simulink model "Quaternions_Method_merge"  (R2021b)
settings: Solver=VariableStepAuto  StartTime=0.0  StopTime=Time  MinStep=1e-3  RelTol=1e-13  AbsTol=1e-8
undefined symbols (not defined in the file): a, c, e, f_mag, H_0, i, magnitude, MB, muP, omega_0, p_acc, RD, RS_MB, RS_SP, SP, theta0, w_E
libraries: matrix_library x10, vrlib x4, simulink_extras x1
(part 1 of 3)
settings Model: Creator=dario  LastModifiedBy=hp
settings SolverCC: ZeroCrossControl=DisableAll  ZeroCrossAlgorithm=Adaptive  AlgebraicLoopSolver=TrustRegion
settings DebuggingCC: IgnoredZcDiagnostic=none

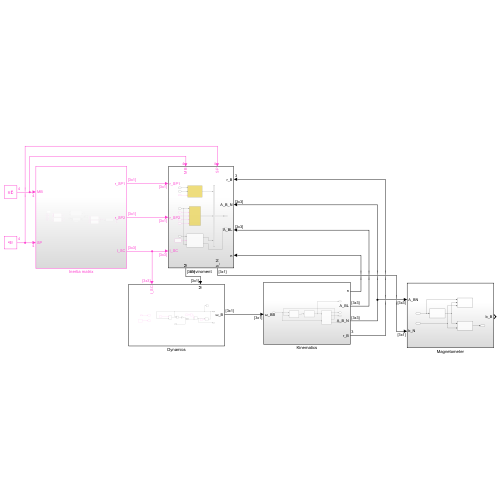
[thumbnail: Simulink's stored preview of the top-level diagram]
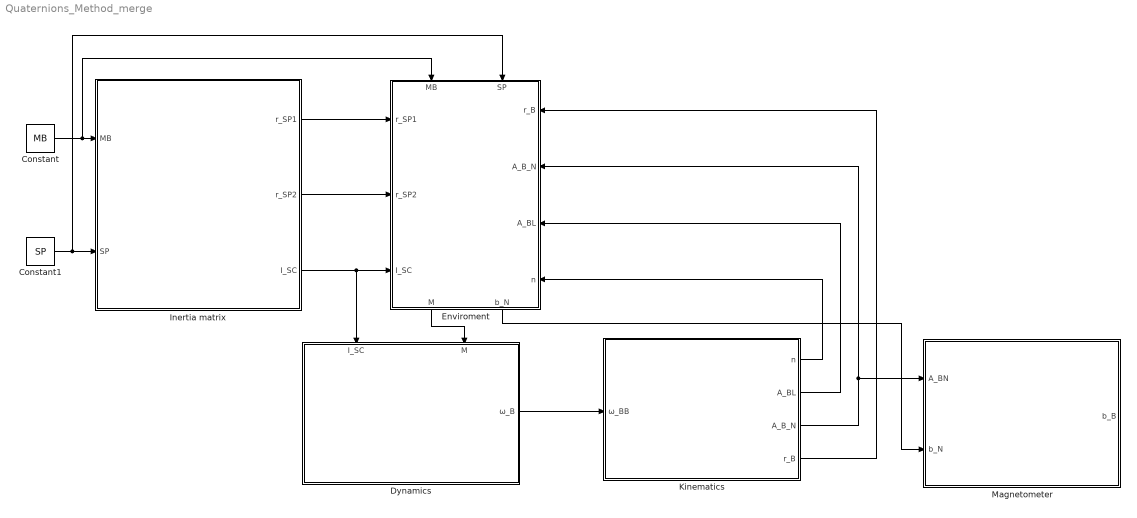
== system Quaternions_Method_merge ==
  Constant : Constant  Value=MB
  Constant1 : Constant  Value=SP
  Dynamics : Subsystem
      settings: PortSchema="{\"entries\":[{\"content\":{\"sides\":[{\"content\":{\"connectorIds\":[]},\"type\":\"ConnectorPlacement.EquallySpacedRectSide\",\"uuid\":\"0fb0fd28-732a-45b7-951f-4b0b2306202c\"},{\"content\":{\"connectorIds\":[\"Out1\"],\"side\":\"RIGHT\"},\"type\":\"ConnectorPlacement.EquallySpacedRectSide\",\"uuid\":\"160a6d95-5e8b-4088-9ac4-372e2ef53b1e\"},{\"content\":{\"connectorIds\":[\"In1\",\"In2\"],\"side\":\"TOP\"},\"type\":\"ConnectorPlacement.EquallySpacedRectSide\",\"uuid\":\"bc0d773d-9b3c-40c2-804a-fc9efd6e220c\"}]},\"type\":\"ConnectorPlacement.EquallySpacedConnector\",\"uuid\":\"1f85a25c-c8d4-4d9d-9994-483d99135538\"}],\"packageUris\":[\"http://schema.mathworks.com/mf0/Connector/R2020b\"],\"version\":\"1.0\"}"
  Enviroment : Subsystem
      settings: PortSchema="{\"entries\":[{\"content\":{\"sides\":[{\"content\":{\"connectorIds\":[\"In1\",\"In2\"]},\"type\":\"ConnectorPlacement.EquallySpacedRectSide\",\"uuid\":\"77a65197-c5ef-4c05-af97-bd670bb59a1b\"},{\"content\":{\"connectorIds\":[\"Out1\",\"Out2\"],\"side\":\"RIGHT\"},\"type\":\"ConnectorPlacement.EquallySpacedRectSide\",\"uuid\":\"f4905732-994b-44e8-915f-1f1165b6d340\"},{\"content\":{\"connectorIds\":[\"In3\",\"In4\",\"In5\"],\"side\":\"TOP\"},\"type\":\"ConnectorPlacement.EquallySpacedRectSide\",\"uuid\":\"dbb628bc-072b-4daa-a580-a056bf799753\"},{\"content\":{\"connectorIds\":[\"In6\",\"In7\",\"In8\",\"In9\"],\"side\":\"BOTTOM\"},\"type\":\"ConnectorPlacement.EquallySpacedRectSide\",\"uuid\":\"e6af6235-b92e-4098-9bbc-91b77f168ead\"}]},\"type\":\"ConnectorPlacement.EquallySpacedConnector\",\"uuid\":\"a4645f0d-8f51-4ba7-9ec5-d423e83ccc17\"}],\"packageUris\":[\"http://schema.mathworks.com/mf0/Connector/R2020b\"],\"version\":\"1.0\"}"
  Inertia matrix : Subsystem
  Kinematics : Subsystem
  Magnetometer : Subsystem
  wires:
  Enviroment/1(M) -> Dynamics/2(M)
  Kinematics/2(A_BL) -> Enviroment/8(A_BL)
  Dynamics/1(ω_B) -> Kinematics/1(ω_BB)
  Kinematics/1(n) -> Enviroment/9(n)
  Kinematics/3(A_B_N) -> Magnetometer/1(A_BN), Enviroment/7(A_B_N)
  Constant/1 -> Inertia matrix/1(MB), Enviroment/1(MB)
  Constant1/1 -> Inertia matrix/2(SP), Enviroment/2(SP)
  Inertia matrix/1(r_SP1) -> Enviroment/3(r_SP1)
  Inertia matrix/2(r_SP2) -> Enviroment/4(r_SP2)
  Inertia matrix/3(I_SC) -> Dynamics/1(I_SC), Enviroment/5(I_SC)
  Kinematics/4(r_B) -> Enviroment/6(r_B)
  Enviroment/2(b_N) -> Magnetometer/2(b_N)

== system Quaternions_Method_merge/Dynamics ==
  I_SC : Inport
  M : Inport  Port=2
  Constant7 : Constant  Value=omega_0
  Cross Product : vrlib/Utilities/Cross Product
  Gain5 : Gain  Gain=-1
  Integrator4 : Integrator  InitialConditionSource=external  InitialCondition=omega_0
  Product6 : Product  Multiplication=Matrix(*)
  Product7 : Product  Multiplication=Matrix(*)
  Reciprocal : Product  Inputs=/  Multiplication=Matrix(*)
  Scope : Scope
  Sum2 : Sum
  Terminator : Terminator
  ω_B : Outport
  wires:
  Sum2/1 -> Product7/2
  Product6/1 -> Cross Product/2
  Product7/1 -> Terminator/1, Integrator4/1
  Cross Product/1 -> Gain5/1
  Gain5/1 -> Sum2/1
  Integrator4/1 -> Scope/1, Cross Product/1, Product6/2, ω_B/1
  I_SC/1 -> [I_SC]
  [I_SC] -> Product6/1
  [I_SC] -> Reciprocal/1
  Reciprocal/1 -> Product7/1
  Constant7/1 -> [w_0]
  [w_0] -> Integrator4/2
  M/1 -> Sum2/2

== system Quaternions_Method_merge/Enviroment ==
  MB : Inport
  SP : Inport  Port=2
  r_SP1 : Inport  Port=3
  r_SP2 : Inport  Port=4
  I_SC : Inport  Port=5
  r_B : Inport  Port=6
  A_B_N : Inport  Port=7
  A_BL : Inport  Port=8
  n : Inport  Port=9
  Constant : Constant  Value=6371.2*1e3
  Gravity Gradient : Subsystem
  "Magnetic torque " : Subsystem
  Solar Radiation Perturbation : Subsystem
  Sum : Sum  Inputs=+|+|+
  M : Outport
  b_N : Outport  Port=2
  wires:
  A_BL/1 -> Gravity Gradient/1(A_BL)
  n/1 -> Gravity Gradient/2(n)
  A_B_N/1 -> "Magnetic torque "/3(A_B_N), Solar Radiation Perturbation/1(A_B_N)
  MB/1 -> Solar Radiation Perturbation/2(MB)
  SP/1 -> Solar Radiation Perturbation/3(SP)
  r_SP1/1 -> Solar Radiation Perturbation/4(r_SP1)
  r_SP2/1 -> Solar Radiation Perturbation/5(r_SP2)
  Sum/1 -> M/1
  Gravity Gradient/1(M_GG) -> Sum/1
  Solar Radiation Perturbation/1(M_SRP) -> Sum/2
  I_SC/1 -> Gravity Gradient/3(I_SC)
  "Magnetic torque "/1(M) -> Sum/3
  r_B/1 -> "Magnetic torque "/1(r_B)
  Constant/1 -> "Magnetic torque "/2(R)
  "Magnetic torque "/2(b_N) -> b_N/1

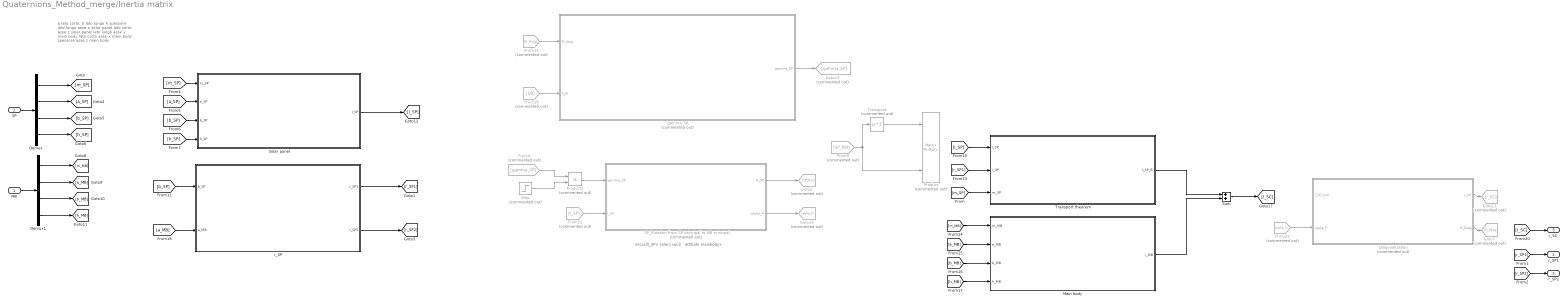
== system Quaternions_Method_merge/Inertia matrix ==
  note: arcos(S_B*n solary)-pi/2 - attitude mainbodyx
  note: a lato corto, b lato lungo h spessore
      | lato lungo asse x solar panel
      | lato corto asse z solar panel
      | lato lungo asse y main body
      | lato corto asse x main body
      | spessore asse z main body
  MB : Inport
  SP : Inport  Port=2
  Demux : Demux
  Demux1 : Demux
  Diagonalization : Subsystem  Commented=on
  From12 : From  Commented=on  GotoTag=R_Diag
  From19 : From  Commented=on  GotoTag=SB
  From21 : From  Commented=on  GotoTag=I_SP
  From22 : From  Commented=on  GotoTag=alpha_P
  From8 : From  Commented=on  GotoTag=gamma_SP
  From9 : From  Commented=on  GotoTag=SP_Rot
  Goto13 : Goto  Commented=on  GotoTag=I_SC
  Goto14 : Goto  Commented=on  GotoTag=gamma_SP
  Goto16 : Goto  Commented=on  GotoTag=alpha_P
  Goto2 : Goto  Commented=on  GotoTag=SP_Rot
  Goto7 : Goto  Commented=on  GotoTag=R_Diag
  Main body : Subsystem
  Product : Product  Commented=on  Inputs=3  Multiplication=Matrix(*)
  Product1 : Product  Commented=on
  SP_Rotation from SP principal to MB principal : Subsystem  Commented=on
  Solar panel : Subsystem
  Step : Step  Commented=on  Time=1e-3  SampleTime=0
  Sum : Sum
  Transport theorem : Subsystem
  Transpose : Math  Commented=on  Operator=transpose  SaturateOnIntegerOverflow=on
  gamma_SP : Subsystem  Commented=on
  r_SP : Subsystem
  r_SP1 : Outport
  r_SP2 : Outport  Port=2
  I_SC : Outport  Port=3
  wires:
  MB/1 -> Demux1/1
  Demux/1 -> [m_SP]
  SP_Rotation from SP principal to MB principal/1(R_SP) -> Goto2/1
  Transpose/1 -> Product/1
  Transport theorem/1(I_SP_B) -> Sum/1
  [r_SP1] -> Transport theorem/2(r_SP)
  Main body/1(I_MB) -> Sum/2
  [m_SP] -> Transport theorem/3(m_SP)
  r_SP/1(r_SP1) -> [r_SP1]
  [r_SP1] -> r_SP1/1
  [r_SP2] -> r_SP2/1
  r_SP/2(r_SP2) -> [r_SP2]
  Demux/2 -> [a_SP]
  Demux/3 -> [b_SP]
  Demux/4 -> [h_SP]
  [a_SP] -> Solar panel/2(a_SP)
  [b_SP] -> Solar panel/3(b_SP)
  [m_SP] -> Solar panel/1(m_SP)
  [h_SP] -> Solar panel/4(h_SP)
  From9/1 -> Transpose/1, Product/3
  [b_SP] -> r_SP/1(b_SP)
  Demux1/4 -> [h_MB]
  Demux1/3 -> [b_MB]
  Demux1/2 -> [a_MB]
  Demux1/1 -> [m_MB]
  [m_MB] -> Main body/1(m_MB)
  [a_MB] -> Main body/2(a_MB)
  [b_MB] -> Main body/3(b_MB)
  [h_MB] -> Main body/4(h_MB)
  [a_MB] -> r_SP/2(a_MB)
  Solar panel/1(I_SP) -> [I_SP]
  Product1/1 -> SP_Rotation from SP principal to MB principal/1(gamma_SP)
  From8/1 -> Product1/1
  Step/1 -> Product1/2
  SP/1 -> Demux/1
  Diagonalization/2(R_Diag) -> Goto7/1
  From12/1 -> gamma_SP/1(R_diag)
  From19/1 -> gamma_SP/2(S_B)
  Diagonalization/1(I_SC) -> Goto13/1
  [I_SC] -> I_SC/1
  gamma_SP/1(gamma_SP) -> Goto14/1
  From21/1 -> SP_Rotation from SP principal to MB principal/2(I_SP)
  SP_Rotation from SP principal to MB principal/2(alpha_P) -> Goto16/1
  From22/1 -> Diagonalization/2(alpha_P)
  [I_SP] -> Transport theorem/1(I_SP)
  Sum/1 -> [I_SC]

== system Quaternions_Method_merge/Kinematics ==
  ω_BB : Inport
  Creazione Matrice A_BN : Subsystem
  Creazione quaternione : Subsystem
  Relative_Attitude : Subsystem
  n : Outport
  A_BL : Outport  Port=2
  A_B_N : Outport  Port=3
  r_B : Outport  Port=4
  wires:
  Creazione Matrice A_BN/1(A_BN) -> A_B_N/1, Relative_Attitude/1(A_BN)
  ω_BB/1 -> Creazione quaternione/1(ω_BB), Relative_Attitude/2(ω_BB)
  Creazione quaternione/1(q_normalizzato) -> Creazione Matrice A_BN/1(q_normalizzato)
  Relative_Attitude/1(A_BL) -> A_BL/1
  Relative_Attitude/2(n) -> n/1
  Relative_Attitude/3(A_L/N) -> Creazione quaternione/2(A_LN)
  Relative_Attitude/4(r_B) -> r_B/1

== system Quaternions_Method_merge/Magnetometer ==
  A_BN : Inport
  b_N : Inport  Port=2
  Compute b_B : Subsystem
  Difference between model and reality : Subsystem
  "Magnetometer " : Subsystem
  b_B : Outport
  wires:
  "Magnetometer "/1(A_BN*) -> Compute b_B/1(A_BN*), Difference between model and reality/2(A_BN*)
  A_BN/1 -> Difference between model and reality/1(A_BN), "Magnetometer "/1(A_BN)
  b_N/1 -> Compute b_B/2(b_N), Difference between model and reality/3(b_N)
  Compute b_B/1(b_B) -> b_B/1

== system Quaternions_Method_merge/Enviroment/Gravity Gradient ==
  A_BL : Inport
  n : Inport  Port=2
  I_SC : Inport  Port=3
  Constant1 : Constant  Value=[1; 0; 0]
  Demux : Demux  Outputs=9
  Demux2 : Demux  Outputs=3
  Gain1 : Gain  Gain=3
  Matrix Multiply : Product  Multiplication=Matrix(*)
  Mux1 : Mux  Inputs=3
  Product{,4..11} (9 alike) : Product
  Reshape : Reshape  OutputDimensionality=Column vector (2-D)
  Reshape1 : Reshape  OutputDimensionality=Column vector (2-D)
  Square1 : Math  Operator=square  SaturateOnIntegerOverflow=on
  Sum3 : Sum  Inputs=|+|-|
  Sum4 : Sum  Inputs=|+|-|
  Sum5 : Sum  Inputs=|+|-|
  Terminator{,1..5} (6 alike) : Terminator
  M_GG : Outport
  wires:
  A_BL/1 -> Matrix Multiply/1
  Constant1/1 -> Matrix Multiply/2
  Matrix Multiply/1 -> Demux2/1
  Demux2/1 -> Product4/1, Product/1  "c1"
  Demux2/3 -> Product5/2, Product4/2  "c3"
  Demux2/2 -> Product5/1, Product/2  "c2"
  Demux/9 -> Sum4/2, Sum3/1  "Iz"
  Demux/5 -> Sum5/1, Sum3/2  "Iy"
  Demux/1 -> Sum5/2, Sum4/1  "Ix"
  n/1 -> Square1/1
  Square1/1 -> Gain1/1
  Product5/1 -> Product6/1
  Gain1/1 -> Product9/2, Product7/2, Product6/2
  Product4/1 -> Product7/1
  Product/1 -> Product9/1
  Sum3/1 -> Product8/1
  Product6/1 -> Product8/2
  Product7/1 -> Product10/1
  Sum4/1 -> Product10/2
  Sum5/1 -> Product11/2
  Product9/1 -> Product11/1
  Product10/1 -> Mux1/2
  Product8/1 -> Mux1/1
  Product11/1 -> Mux1/3
  Mux1/1 -> Reshape/1
  Reshape/1 -> M_GG/1
  I_SC/1 -> Reshape1/1
  Demux/2 -> Terminator/1
  Demux/3 -> Terminator1/1
  Demux/4 -> Terminator2/1
  Demux/6 -> Terminator3/1
  Demux/7 -> Terminator4/1
  Demux/8 -> Terminator5/1
  Reshape1/1 -> Demux/1

== system Quaternions_Method_merge/Enviroment/Magnetic torque  ==
  r_B : Inport
  R : Inport  Port=2
  A_B_N : Inport  Port=3
  Creation of parasitic torque : Subsystem
  Magnetic torque in body frame : Subsystem
  Matrix Multiply : Product  Multiplication=Matrix(*)
  Product : Product
  M : Outport
  b_N : Outport  Port=2
  wires:
  R/1 -> Magnetic torque in body frame/3(R)
  A_B_N/1 -> Magnetic torque in body frame/1(A_B_N), Matrix Multiply/1
  Magnetic torque in body frame/1(b_B) -> Product/1
  Creation of parasitic torque/1(m) -> Product/2
  Product/1 -> M/1
  Matrix Multiply/1 -> Magnetic torque in body frame/2(r_N)
  r_B/1 -> Matrix Multiply/2
  Magnetic torque in body frame/2(b_N) -> b_N/1

== system Quaternions_Method_merge/Enviroment/Solar Radiation Perturbation ==
  A_B_N : Inport
  MB : Inport  Port=2
  SP : Inport  Port=3
  r_SP1 : Inport  Port=4
  r_SP2 : Inport  Port=5
  Force : Subsystem
  Normalize Vector : vrlib/Utilities/Normalize Vector  maxzero=0
  Sum forces : Subsystem
      settings: PortSchema="{\"entries\":[{\"content\":{\"sides\":[{\"content\":{\"connectorIds\":[\"In1\",\"In2\",\"In3\",\"In4\",\"In5\",\"In6\",\"In7\"]},\"type\":\"ConnectorPlacement.EquallySpacedRectSide\",\"uuid\":\"5acb7d4f-0337-4224-9758-4598a3a00165\"},{\"content\":{\"connectorIds\":[\"Out1\"],\"side\":\"RIGHT\"},\"type\":\"ConnectorPlacement.EquallySpacedRectSide\",\"uuid\":\"e6f98c05-9b5f-4378-b9e9-dabff353d596\"},{\"content\":{\"connectorIds\":[],\"side\":\"TOP\"},\"type\":\"ConnectorPlacement.EquallySpacedRectSide\",\"uuid\":\"88e90ea7-7ab4-48d4-8e3b-8712b3a0b993\"},{\"content\":{\"connectorIds\":[\"In8\"],\"side\":\"BOTTOM\"},\"type\":\"ConnectorPlacement.EquallySpacedRectSide\",\"uuid\":\"ececea6a-2c27-462e-a638-503b4beb3cbf\"}]},\"type\":\"ConnectorPlacement.EquallySpacedConnector\",\"uuid\":\"86da1db6-5ce7-4d9e-9b5c-c43957a7360d\"}],\"packageUris\":[\"http://schema.mathworks.com/mf0/Connector/R2020b\"],\"version\":\"1.0\"}"
  Sun position body : Subsystem
  normali SP1 : Constant  Value=[0 1 0; 0 -1 0; 0 1 0; 0 -1 0]
  M_SRP : Outport
  tag scope: S_B=global
  wires:
  A_B_N/1 -> Sun position body/1(A_B_N)
  Sun position body/1(S_B) -> Normalize Vector/1
  Normalize Vector/1 -> [S_B], Force/1(SB)
  Force/3(A_MB) -> Sum forces/5(A_MB)
  Force/1(F_MB) -> Sum forces/3(F_MB)
  normali SP1/1 -> Force/2(N_SP)
  r_SP1/1 -> Sum forces/1(r_SP1)
  r_SP2/1 -> Sum forces/2(r_SP2)
  Force/5(prodscal_SP) -> Sum forces/7(prodscal_SP (tra norm e sun direction))
  Force/4(prodsca_MB) -> Sum forces/6(prodscal_MB(tra norm e sun direction))
  Sum forces/1(M_SRP) -> M_SRP/1
  MB/1 -> [MB]
  SP/1 -> [SP]
  [MB] -> Force/3(MB)
  [SP] -> Force/4(SP)
  [MB] -> Sum forces/8(MB)
  Force/2(F_SP) -> Sum forces/4(F_SP)

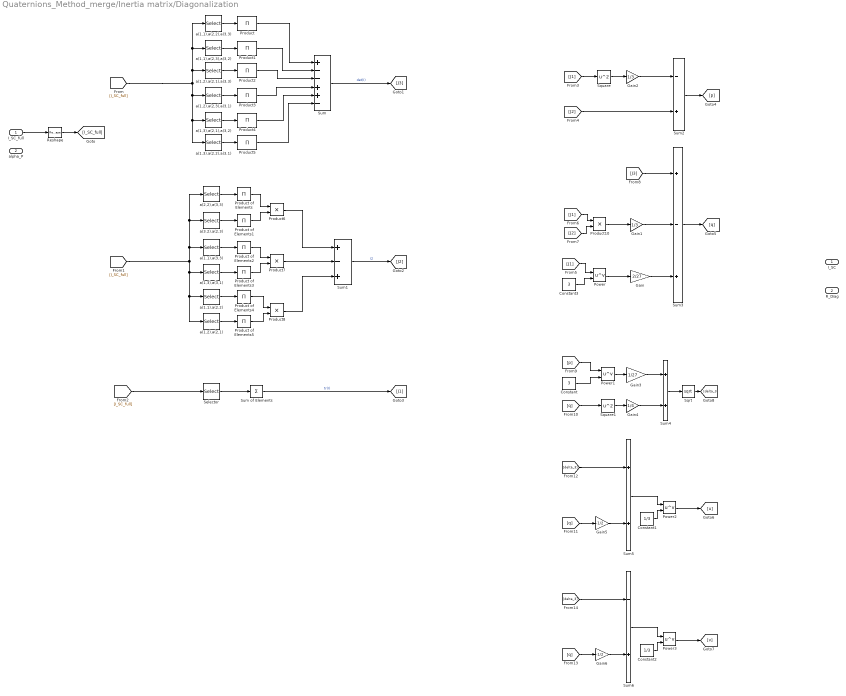
== system Quaternions_Method_merge/Inertia matrix/Diagonalization ==
  I_SC_full : Inport
  alpha_P : Inport  Port=2
  Constant : Constant  Value=3
  Constant1 : Constant  Value=1/3
  Constant2 : Constant  Value=1/3
  Constant3 : Constant  Value=3
  Gain : Gain  Gain=2/27
  Gain1 : Gain  Gain=1/3
  Gain2 : Gain  Gain=1/3
  Gain3 : Gain  Gain=1/27
  Gain4 : Gain  Gain=1/4
  Gain5 : Gain  Gain=-1/2
  Gain6 : Gain  Gain=-1/2
  Power{,1..3} (4 alike) : Math  Operator=pow  SaturateOnIntegerOverflow=on
  Product{,1..5} (6 alike) : Product  Inputs=1  SaturateOnIntegerOverflow=on  OutDataTypeStr=Inherit: Same as first input
  Product of Elements{,1..5} (6 alike) : Product  Inputs=*
  Product{6..8,10} (4 alike) : Product
  Reshape : Reshape  OutputDimensionality=Column vector (2-D)
  Selector : Selector  InputPortWidth=9  IndexOptions=Index vector (dialog)  Indices=[1 5 9]  OutputSizes=1
  Sqrt : Sqrt  SaturateOnIntegerOverflow=on
  Square : Math  Operator=square  SaturateOnIntegerOverflow=on
  Square1 : Math  Operator=square  SaturateOnIntegerOverflow=on
  Sum : Sum  Inputs=+--++-  SaturateOnIntegerOverflow=on
  Sum of Elements : Sum  Inputs=+
  Sum1 : Sum  Inputs=+-+
  Sum2 : Sum  Inputs=-+
  Sum3 : Sum  Inputs=+-+
  Sum4 : Sum
  Sum5 : Sum
  Sum6 : Sum  Inputs=-+
  a(1,1),a(2,2) : Selector  InputPortWidth=9  IndexOptions=Index vector (dialog)  Indices=[1 3]  OutputSizes=1
  a(1,1),a(2,2),a(3,3) : Selector  InputPortWidth=9  IndexOptions=Index vector (dialog)  Indices=[1 5 9]  OutputSizes=1
  a(1,1),a(2,3),a(3,2) : Selector  InputPortWidth=9  IndexOptions=Index vector (dialog)  Indices=[1 6 8]  OutputSizes=1
  a(1,2),a(2,1) : Selector  InputPortWidth=9  IndexOptions=Index vector (dialog)  Indices=[1 3]  OutputSizes=1
  a(1,2),a(2,1),a(3,3) : Selector  InputPortWidth=9  IndexOptions=Index vector (dialog)  Indices=[2 4 9]  OutputSizes=1
  a(1,2),a(2,3),a(3,1) : Selector  InputPortWidth=9  IndexOptions=Index vector (dialog)  Indices=[3 4 8]  OutputSizes=1
  a(1,3),a(2,1),a(3,2) : Selector  InputPortWidth=9  IndexOptions=Index vector (dialog)  Indices=[2 6 7]  OutputSizes=1
  a(1,3),a(2,2),a(3,1) : Selector  InputPortWidth=9  IndexOptions=Index vector (dialog)  Indices=[3 5 7]  OutputSizes=1
  a(1,3),a(3,1) : Selector  InputPortWidth=9  IndexOptions=Index vector (dialog)  Indices=[1 3]  OutputSizes=1
  a(1.1),a(3,3) : Selector  InputPortWidth=9  IndexOptions=Index vector (dialog)  Indices=[1 3]  OutputSizes=1
  a(2,2),a(3,3) : Selector  InputPortWidth=9  IndexOptions=Index vector (dialog)  Indices=[5 9]  OutputSizes=1
  a(3.2),a(2,3) : Selector  InputPortWidth=9  IndexOptions=Index vector (dialog)  Indices=[6 8]  OutputSizes=1
  I_SC : Outport
  R_Diag : Outport  Port=2
  wires:
  [I_SC_full] -> a(1,3),a(2,2),a(3,1)/1, a(1,3),a(2,1),a(3,2)/1, a(1,2),a(2,3),a(3,1)/1, a(1,1),a(2,2),a(3,3)/1, a(1,1),a(2,3),a(3,2)/1, a(1,2),a(2,1),a(3,3)/1
  Product2/1 -> Sum/3
  Product3/1 -> Sum/4
  a(1,2),a(2,1),a(3,3)/1 -> Product2/1
  a(1,1),a(2,3),a(3,2)/1 -> Product1/1
  Product/1 -> Sum/1
  a(1,3),a(2,2),a(3,1)/1 -> Product5/1
  a(1,1),a(2,2),a(3,3)/1 -> Product/1
  a(1,3),a(2,1),a(3,2)/1 -> Product4/1
  Product4/1 -> Sum/5
  Product1/1 -> Sum/2
  Product5/1 -> Sum/6
  a(1,2),a(2,3),a(3,1)/1 -> Product3/1
  I_SC_full/1 -> Reshape/1
  Reshape/1 -> [I_SC_full]
  Sum/1 -> [J3]  "det(I)"
  Product6/1 -> Sum1/1
  Product7/1 -> Sum1/2
  Product8/1 -> Sum1/3
  Sum1/1 -> [J2]  "I2"
  [I_SC_full] -> a(1,3),a(3,1)/1, a(1,1),a(2,2)/1, a(1,2),a(2,1)/1, a(1.1),a(3,3)/1, a(3.2),a(2,3)/1, a(2,2),a(3,3)/1
  [I_SC_full] -> Selector/1
  Selector/1 -> Sum of Elements/1
  a(2,2),a(3,3)/1 -> Product of Elements/1
  a(3.2),a(2,3)/1 -> Product of Elements1/1
  a(1.1),a(3,3)/1 -> Product of Elements2/1
  a(1,3),a(3,1)/1 -> Product of Elements3/1
  a(1,1),a(2,2)/1 -> Product of Elements4/1
  a(1,2),a(2,1)/1 -> Product of Elements5/1
  Product of Elements5/1 -> Product8/2
  Product of Elements4/1 -> Product8/1
  Product of Elements3/1 -> Product7/2
  Product of Elements2/1 -> Product7/1
  Product of Elements1/1 -> Product6/2
  Product of Elements/1 -> Product6/1
  Sum of Elements/1 -> [J1]  "tr(I)"
  [J2] -> Sum2/2
  [J1] -> Square/1
  Square/1 -> Gain2/1
  Gain2/1 -> Sum2/1
  Sum2/1 -> [p]
  [J2] -> Product10/2
  [J1] -> Product10/1
  [J3] -> Sum3/1
  Constant3/1 -> Power/2
  [J1] -> Power/1
  Power/1 -> Gain/1
  Product10/1 -> Gain1/1
  Gain1/1 -> Sum3/2
  Gain/1 -> Sum3/3
  Sum3/1 -> [q]
  [q] -> Square1/1
  [p] -> Power1/1
  Constant/1 -> Power1/2
  Square1/1 -> Gain4/1
  Power1/1 -> Gain3/1
  Gain4/1 -> Sum4/2
  Gain3/1 -> Sum4/1
  Sum4/1 -> Sqrt/1
  [q] -> Gain5/1
  Gain5/1 -> Sum5/2
  Sum5/1 -> Power2/1
  Constant1/1 -> Power2/2
  Power2/1 -> [u]
  Sqrt/1 -> [delta_3]
  [delta_3] -> Sum5/1
  [delta_3] -> Sum6/1
  Constant2/1 -> Power3/2
  Sum6/1 -> Power3/1
  [q] -> Gain6/1
  Power3/1 -> [v]
  Gain6/1 -> Sum6/2

== system Quaternions_Method_merge/Inertia matrix/Main body ==
  m_MB : Inport
  a_MB : Inport  Port=2
  b_MB : Inport  Port=3
  h_MB : Inport  Port=4
  Constant : Constant  Value=0
  Gain : Gain  Gain=1/12
  Gain1 : Gain  Gain=1/12
  Gain2 : Gain  Gain=1/12
  Product : Product
  Product1 : Product
  Product2 : Product
  Reshape : Reshape  OutputDimensionality=Customize  OutputDimensions=[3,3]
  Square : Math  Operator=square  SaturateOnIntegerOverflow=on
  Square1 : Math  Operator=square  SaturateOnIntegerOverflow=on
  Square2 : Math  Operator=square  SaturateOnIntegerOverflow=on
  Sum : Sum
  Sum1 : Sum
  Sum2 : Sum
  Vector Concatenate : Concatenate  NumInputs=9
  I_MB : Outport
  wires:
  Constant/1 -> Vector Concatenate/2, Vector Concatenate/3, Vector Concatenate/7, Vector Concatenate/8, Vector Concatenate/6, Vector Concatenate/4
  Square/1 -> Sum2/1, Sum1/1
  Square1/1 -> Sum2/2, Sum/1
  Square2/1 -> Sum/2, Sum1/2
  Product1/1 -> Gain1/1
  Gain/1 -> Vector Concatenate/1
  Product2/1 -> Gain2/1
  Sum1/1 -> Product1/2
  m_MB/1 -> Product/1, Product2/1, Product1/1
  Sum2/1 -> Product2/2
  a_MB/1 -> Square/1
  Vector Concatenate/1 -> Reshape/1
  Sum/1 -> Product/2
  b_MB/1 -> Square1/1
  Gain1/1 -> Vector Concatenate/5
  Product/1 -> Gain/1
  Gain2/1 -> Vector Concatenate/9
  Reshape/1 -> I_MB/1
  h_MB/1 -> Square2/1

== system Quaternions_Method_merge/Inertia matrix/SP_Rotation from SP principal to MB principal ==
  gamma_SP : Inport
  I_SP : Inport  Port=2
  Constant : Constant
  Demux : Demux  Outputs=9
  Gain : Gain  Gain=-1
  Gain1 : Gain  Gain=2
  Gain2 : Gain  Gain=1/2
  Ground : Ground
  Product : Product
  Reciprocal : Product  Inputs=/
  Reshape : Reshape  OutputDimensionality=Customize  OutputDimensions=[3,3]
  Sin : Trigonometry  Operator=cos
  Sin1 : Trigonometry
  Sin2 : Trigonometry  Operator=atan
  Sum : Sum  Inputs=+-
  Sum1 : Sum
  Terminator{,1..5} (6 alike) : Terminator
  Vector Concatenate : Concatenate  NumInputs=9
  R_SP : Outport
  alpha_P : Outport  Port=2
  wires:
  Vector Concatenate/1 -> Reshape/1
  Reshape/1 -> R_SP/1
  Constant/1 -> Vector Concatenate/1
  Ground/1 -> Vector Concatenate/7, Vector Concatenate/4, Vector Concatenate/3, Vector Concatenate/2
  gamma_SP/1 -> Sum1/1
  Gain/1 -> Vector Concatenate/6
  Sin/1 -> Vector Concatenate/5, Vector Concatenate/9
  Sin1/1 -> Gain/1, Vector Concatenate/8
  I_SP/1 -> Demux/1
  Demux/1 -> Terminator/1
  Demux/2 -> Terminator1/1
  Demux/3 -> Terminator2/1
  Demux/4 -> Terminator3/1
  Demux/5 -> Sum/1  "I22"
  Demux/6 -> Gain1/1  "I31"
  Demux/7 -> Terminator4/1
  Demux/8 -> Terminator5/1
  Demux/9 -> Sum/2  "I33"
  Sum/1 -> Reciprocal/1
  Reciprocal/1 -> Product/1
  Gain1/1 -> Product/2
  Product/1 -> Sin2/1
  Sin2/1 -> Gain2/1
  Gain2/1 -> alpha_P/1, Sum1/2
  Sum1/1 -> Sin1/1, Sin/1

== system Quaternions_Method_merge/Inertia matrix/Solar panel ==
  note: The inertia matrix for the solar panels is for two solar panels since they are the same and they are on opposite sides the distance vector between the centers of mass are one the opposite of the other and in the transport theorem the sign does not matter since I need only the norm and the d'*d that has + sign anyway
      | Still the mass and all characteristics are about one solar panel
  m_SP : Inport
  a_SP : Inport  Port=2
  b_SP : Inport  Port=3
  h_SP : Inport  Port=4
  Gain : Gain  Gain=1/12
  Gain1 : Gain  Gain=1/12
  Gain2 : Gain  Gain=1/12
  Gain3 : Gain  Gain=2
  Ground : Ground
  Product : Product
  Product1 : Product
  Product2 : Product
  Reshape : Reshape  OutputDimensionality=Customize  OutputDimensions=[3,3]
  Square : Math  Operator=square  SaturateOnIntegerOverflow=on
  Square1 : Math  Operator=square  SaturateOnIntegerOverflow=on
  Square2 : Math  Operator=square  SaturateOnIntegerOverflow=on
  Sum : Sum
  Sum1 : Sum
  Sum2 : Sum
  Vector Concatenate : Concatenate  NumInputs=9
  I_SP : Outport
  wires:
  Vector Concatenate/1 -> Reshape/1
  m_SP/1 -> Product/1, Product2/1, Product1/1
  Product/1 -> Gain/1
  Gain/1 -> Vector Concatenate/1
  Product1/1 -> Gain1/1
  Product2/1 -> Gain2/1
  Gain2/1 -> Vector Concatenate/9
  h_SP/1 -> Square/1
  a_SP/1 -> Square1/1
  b_SP/1 -> Square2/1
  Sum/1 -> Product/2
  Sum1/1 -> Product1/2
  Sum2/1 -> Product2/2
  Ground/1 -> Vector Concatenate/2, Vector Concatenate/3, Vector Concatenate/7, Vector Concatenate/8, Vector Concatenate/6, Vector Concatenate/4
  Gain1/1 -> Vector Concatenate/5
  Reshape/1 -> Gain3/1
  Gain3/1 -> I_SP/1
  Square1/1 -> Sum1/2, Sum2/1
  Square2/1 -> Sum/2, Sum2/2
  Square/1 -> Sum/1, Sum1/1

== system Quaternions_Method_merge/Inertia matrix/Transport theorem ==
  I_SP : Inport
  r_SP : Inport  Port=2
  m_SP : Inport  Port=3
  Constant : Constant  Value=eye(3)
  Dot Product : DotProduct  InputSameDT=on  OutDataTypeStr=Inherit: Inherit via internal rule
  Gain : Gain  Gain=2
  Matrix Multiply : Product  Multiplication=Matrix(*)
  Matrix Multiply1 : Product
  Product : Product
  Sum : Sum  Inputs=+-
  Sum1 : Sum
  Transpose : Math  Operator=transpose  SaturateOnIntegerOverflow=on
  I_SP_B : Outport
  wires:
  r_SP/1 -> Transpose/1, Dot Product/2, Dot Product/1, Matrix Multiply/2
  Transpose/1 -> Matrix Multiply/1
  Constant/1 -> Matrix Multiply1/1
  Matrix Multiply1/1 -> Sum/1
  Matrix Multiply/1 -> Sum/2
  Sum/1 -> Product/2
  m_SP/1 -> Gain/1
  Product/1 -> Sum1/2
  I_SP/1 -> Sum1/1
  Sum1/1 -> I_SP_B/1
  Dot Product/1 -> Matrix Multiply1/2
  Gain/1 -> Product/1

== system Quaternions_Method_merge/Inertia matrix/gamma_SP ==
  R_diag : Inport
  S_B : Inport  Port=2
  Cos : Trigonometry  Operator=acos
  Demux : Demux  Outputs=3
  Gain : Gain  Gain=-1
  Matrix Multiply1 : Product  Multiplication=Matrix(*)
  Terminator : Terminator
  Terminator1 : Terminator
  gamma_SP : Outport
  wires:
  R_diag/1 -> Matrix Multiply1/1
  S_B/1 -> Matrix Multiply1/2
  Matrix Multiply1/1 -> Demux/1  "S_p_SP"
  Demux/1 -> Terminator/1
  Demux/2 -> Terminator1/1
  Demux/3 -> Gain/1
  Gain/1 -> Cos/1
  Cos/1 -> gamma_SP/1

== system Quaternions_Method_merge/Inertia matrix/r_SP ==
  b_SP : Inport
  a_MB : Inport  Port=2
  Constant : Constant  Value=[1 0 0]
  Gain : Gain  Gain=1/2
  Gain1 : Gain  Gain=1/2
  Gain2 : Gain  Gain=-1
  Product : Product
  Reshape : Reshape  OutputDimensionality=Column vector (2-D)
  Sum : Sum
  r_SP1 : Outport
  r_SP2 : Outport  Port=2
  wires:
  Constant/1 -> Reshape/1
  a_MB/1 -> Gain/1
  b_SP/1 -> Gain1/1
  Gain1/1 -> Sum/1
  Gain/1 -> Sum/2
  Reshape/1 -> Product/1
  Sum/1 -> Product/2
  Gain2/1 -> r_SP2/1
  Product/1 -> r_SP1/1, Gain2/1

== system Quaternions_Method_merge/Kinematics/Creazione Matrice A_BN ==
  q_normalizzato : Inport
  Matrix Concatenate : Concatenate  NumInputs=3  Mode=Multidimensional array  ConcatenateDimension=2
  Scope : Scope
  column 1 : Subsystem
  column 2 : Subsystem
  column 3 : Subsystem
  A_BN : Outport
  wires:
  Matrix Concatenate/1 -> Scope/1, A_BN/1
  q_normalizzato/1 -> column 3/1(q_normalizzato), column 1/1(q_normalizzato), column 2/1(q_normalizzato)
  column 1/1(Column 1) -> Matrix Concatenate/1
  column 2/1(Column 2) -> Matrix Concatenate/2
  column 3/1(Column 3) -> Matrix Concatenate/3

== system Quaternions_Method_merge/Kinematics/Creazione quaternione ==
  ω_BB : Inport
  A_LN : Inport  Port=2
  Creation matrix [OM] : MATLAB Function  TreatAsAtomicUnit=on
  Demux : Demux  Outputs=3
  Gain : Gain  Gain=0.5
  Initial condition quaternion : Subsystem
  Integrator : Integrator  InitialConditionSource=external  InitialCondition=[0; 0; 0; 1]
  Matrix Multiply : Product  Multiplication=Matrix(*)
  Normalisation : Subsystem
  Reshape : Reshape  OutputDimensionality=Column vector (2-D)
  q_normalizzato : Outport
  wires:
  Creation matrix [OM]/1(OM) -> Gain/1
  Matrix Multiply/1 -> Integrator/1  "dq/dt"
  Gain/1 -> Matrix Multiply/1
  ω_BB/1 -> Demux/1
  Demux/1 -> Creation matrix [OM]/1(om_x)
  Demux/2 -> Creation matrix [OM]/2(om_y)
  Demux/3 -> Creation matrix [OM]/3(om_z)
  Integrator/1 -> Reshape/1  "q(t)"
  Reshape/1 -> Normalisation/1(In1)
  A_LN/1 -> Initial condition quaternion/1(A_LN)
  Initial condition quaternion/1(Output) -> Integrator/2
  Normalisation/1(Out1) -> q_normalizzato/1, Matrix Multiply/2  "q(t)"

== system Quaternions_Method_merge/Kinematics/Relative_Attitude ==
  A_BN : Inport
  ω_BB : Inport  Port=2
  A_LN : Subsystem
  Constant : Constant  Value=0
  MatrixMultiply : Product  Multiplication=Matrix(*)
  MatrixMultiply1 : Product  Multiplication=Matrix(*)
  Mux : Mux  Inputs=3
  Orbit Propagation : Subsystem
  Reshape : Reshape  OutputDimensionality=Column vector (2-D)
  Sum : Sum  Inputs=-+
  To Workspace : ToWorkspace  VariableName=A_BL  SaveFormat=Timeseries  SampleTime=-1
  To Workspace1 : ToWorkspace  VariableName=Omega_BL  SaveFormat=Timeseries  SampleTime=-1
  Transpose : Math  Operator=transpose  SaturateOnIntegerOverflow=on
  A_BL : Outport
  n : Outport  Port=2
  A_L/N : Outport  Port=3
  r_B : Outport  Port=4
  wires:
  Transpose/1 -> MatrixMultiply/2
  MatrixMultiply/1 -> To Workspace/1, A_BL/1, MatrixMultiply1/1  "A_BL"
  A_LN/1(A_LN) -> A_L/N/1, Transpose/1
  A_BN/1 -> MatrixMultiply/1, Orbit Propagation/1(A_BN)
  ω_BB/1 -> Sum/2
  MatrixMultiply1/1 -> Sum/1
  Sum/1 -> To Workspace1/1  "ω_B/L"
  Orbit Propagation/1(n) -> Mux/3, n/1
  Mux/1 -> Reshape/1  "ω_LN"
  Constant/1 -> Mux/2, Mux/1
  Orbit Propagation/3(rB) -> [r_B]
  Orbit Propagation/2(theta) -> A_LN/1(theta)
  Reshape/1 -> MatrixMultiply1/2
  [r_B] -> r_B/1

== system Quaternions_Method_merge/Magnetometer/Compute b_B ==
  A_BN* : Inport
  b_N : Inport  Port=2
  Matrix Multiply : Product  Multiplication=Matrix(*)
  b_B : Outport
  wires:
  A_BN*/1 -> Matrix Multiply/1
  b_N/1 -> Matrix Multiply/2
  Matrix Multiply/1 -> b_B/1

== system Quaternions_Method_merge/Magnetometer/Difference between model and reality ==
  A_BN : Inport
  A_BN* : Inport  Port=2
  b_N : Inport  Port=3
  MatrixMultiply : Product  Multiplication=Matrix(*)
  MatrixMultiply1 : Product  Multiplication=Matrix(*)
  Scope : Scope
  Sum : Sum  Inputs=|-|+|
  wires:
  A_BN*/1 -> MatrixMultiply/1
  b_N/1 -> MatrixMultiply1/2, MatrixMultiply/2
  A_BN/1 -> MatrixMultiply1/1
  MatrixMultiply1/1 -> Sum/1
  MatrixMultiply/1 -> Sum/2
  Sum/1 -> Scope/1

== system Quaternions_Method_merge/Magnetometer/Magnetometer  ==
  A_BN : Inport
  A_NonOrtho : Subsystem
  A_ScaleFactor : Subsystem
  A_eps : Subsystem  Commented=on
  Matrix Multiply : Product  Inputs=3  Multiplication=Matrix(*)
  Ortonormalisation : Subsystem
  A_BN* : Outport
  wires:
  A_BN/1 -> Matrix Multiply/1
  A_NonOrtho/1(A_no) -> Matrix Multiply/2
  Ortonormalisation/1(A*_orto) -> A_BN*/1
  Matrix Multiply/1 -> Ortonormalisation/1(A*)
  A_ScaleFactor/1(A_sf) -> Matrix Multiply/3

== system Quaternions_Method_merge/Enviroment/Magnetic torque /Creation of parasitic torque ==
  Constant : Constant  Value=0.01
  Constant1 : Constant  Value=0.05
  Constant2 : Constant  Value=0.01
  Mux : Mux  Inputs=3
  Reshape : Reshape  OutputDimensionality=Column vector (2-D)
  m : Outport
  wires:
  Constant/1 -> Mux/1
  Constant1/1 -> Mux/2
  Constant2/1 -> Mux/3
  Mux/1 -> Reshape/1
  Reshape/1 -> m/1

== system Quaternions_Method_merge/Enviroment/Magnetic torque /Magnetic torque in body frame ==
  A_B_N : Inport
  r_N : Inport  Port=2
  R : Inport  Port=3
  Add : Sum  Inputs=+++
  Add1 : Sum  Inputs=+|-
  Constant : Constant  Value=3
  Constant1 : Constant  Value=H_0
  Constant2 : Constant  Value=3
  Definition of m vector : Subsystem
  Demux : Demux  Outputs=3
  Divide : Product  Inputs=*/
  Dot Product : DotProduct  InputSameDT=on  OutDataTypeStr=Inherit: Inherit via internal rule
  Gain : Gain  Gain=3
  Math Function : Math  Operator=pow  SaturateOnIntegerOverflow=on
  Math Function1 : Math  Operator=magnitude^2  SaturateOnIntegerOverflow=on
  Math Function2 : Math  Operator=magnitude^2  SaturateOnIntegerOverflow=on
  Math Function3 : Math  Operator=magnitude^2  SaturateOnIntegerOverflow=on
  Math Function4 : Math  Operator=pow  SaturateOnIntegerOverflow=on
  MatrixMultiply : Product  Multiplication=Matrix(*)
  Normalize Vector : vrlib/Utilities/Normalize Vector  maxzero=0
  Product : Product
  Product1 : Product
  Product2 : Product
  Reshape : Reshape  OutputDimensionality=Column vector (2-D)
  Sqrt : Sqrt  SaturateOnIntegerOverflow=on
  b_B : Outport
  b_N : Outport  Port=2
  wires:
  Normalize Vector/1 -> Product1/1, Dot Product/1
  Demux/2 -> Math Function2/1
  Constant1/1 -> Product/2
  Constant/1 -> Math Function4/2
  Demux/1 -> Math Function1/1
  MatrixMultiply/1 -> b_B/1
  Math Function1/1 -> Add/1
  Demux/3 -> Math Function3/1
  Divide/1 -> Product2/1
  Add/1 -> Sqrt/1
  Math Function/1 -> Divide/2
  Product1/1 -> Gain/1
  Math Function3/1 -> Add/3
  Product/1 -> Divide/1
  Definition of m vector/1(m_vect) -> Add1/2, Dot Product/2
  Math Function4/1 -> Product/1
  Add1/1 -> Product2/2
  Math Function2/1 -> Add/2
  Gain/1 -> Add1/1
  Dot Product/1 -> Product1/2
  Product2/1 -> b_N/1, MatrixMultiply/2  "b_N"
  Sqrt/1 -> Math Function/1
  R/1 -> Math Function4/1
  Reshape/1 -> Demux/1
  r_N/1 -> Reshape/1, Normalize Vector/1
  Constant2/1 -> Math Function/2
  A_B_N/1 -> [A_BN]
  [A_BN] -> MatrixMultiply/1

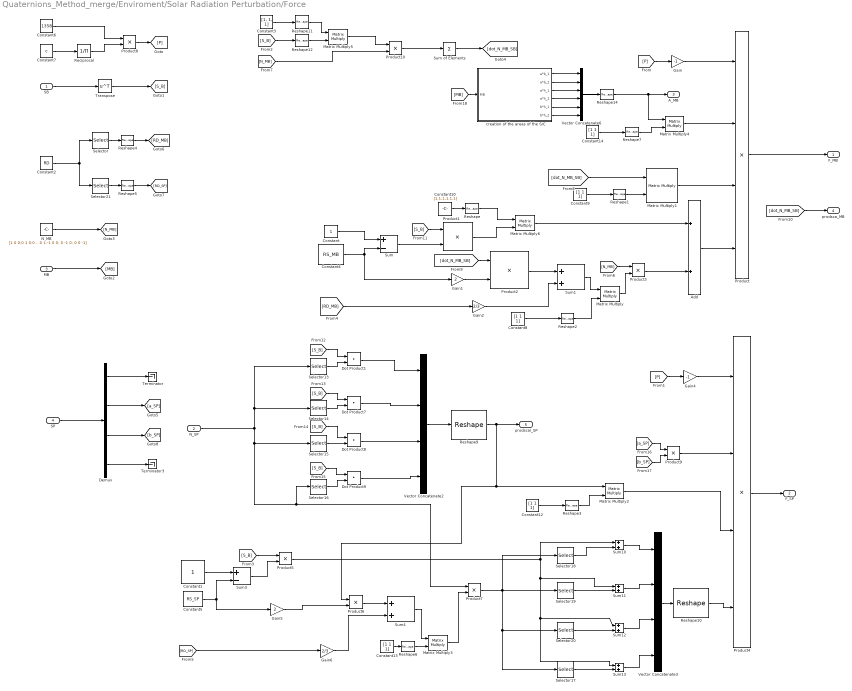
== system Quaternions_Method_merge/Enviroment/Solar Radiation Perturbation/Force ==
  SB : Inport
  N_SP : Inport  Port=2
  MB : Inport  Port=3
  SP : Inport  Port=4
  Add : Sum
  Constant : Constant
  Constant1 : Constant
  Constant10 : Constant  Value=[1,1,1,1,1,1]
  Constant{8..9,12..14} (5 alike) : Constant  Value=[1 1 1]
  Constant2 : Constant  Value=RD
  Constant3 : Constant  Value=[1, 1, 1]
  Constant4 : Constant  Value=RS_MB
  Constant5 : Constant  Value=RS_SP
  Constant6 : Constant  Value=1358
  Constant7 : Constant  Value=c
  Demux : Demux
  Dot Product{1,7..9} (4 alike) : DotProduct  InputSameDT=on  OutDataTypeStr=Inherit: Inherit via internal rule
  Gain : Gain  Gain=-1
  Gain1 : Gain  Gain=2
  Gain2 : Gain  Gain=2/3
  Gain4 : Gain  Gain=-1
  Gain5 : Gain  Gain=2
  Gain6 : Gain  Gain=2/3
  Matrix Multiply{,1..6} (7 alike) : Product  Multiplication=Matrix(*)
  N_MB : Constant  Value=[1 0 0;0 1 0;0 0 1;-1 0 0; 0 -1 0; 0 0 -1]
  Product : Product  Inputs=4
  Product{1..3,5..10} (9 alike) : Product
  Product4 : Product  Inputs=4
  Reciprocal : Product  Inputs=/
  Reshape{,4..5,12,14} (5 alike) : Reshape  OutputDimensionality=Column vector (2-D)
  Reshape{1..3,6..7,11} (6 alike) : Reshape  OutputDimensionality=Row vector (2-D)
  Reshape10 : Reshape  OutputDimensionality=Customize  OutputDimensions=[4,3]
  Reshape9 : Reshape  OutputDimensionality=Customize  OutputDimensions=[4,1]
  Selector : Selector  InputPortWidth=10  IndexOptions=Index vector (dialog)  Indices=[1 2 3 4 5 6]  OutputSizes=1
  Selector13 : Selector  NumberOfDimensions=2  InputPortWidth=3  IndexOptions=Index vector (dialog),Index vector (dialog)  Indices=1,[1 2 3]  OutputSizes=1,1
  Selector14 : Selector  NumberOfDimensions=2  InputPortWidth=3  IndexOptions=Index vector (dialog),Index vector (dialog)  Indices=2,[1 2 3]  OutputSizes=1,1
  Selector15 : Selector  NumberOfDimensions=2  InputPortWidth=3  IndexOptions=Index vector (dialog),Index vector (dialog)  Indices=3,[1 2 3]  OutputSizes=1,1
  Selector16 : Selector  NumberOfDimensions=2  InputPortWidth=3  IndexOptions=Index vector (dialog),Index vector (dialog)  Indices=4,[1 2 3]  OutputSizes=1,1
  Selector17 : Selector  NumberOfDimensions=2  InputPortWidth=3  IndexOptions=Index vector (dialog),Index vector (dialog)  Indices=4,[1 2 3]  OutputSizes=1,1
  Selector18 : Selector  NumberOfDimensions=2  InputPortWidth=3  IndexOptions=Index vector (dialog),Index vector (dialog)  Indices=1,[1 2 3]  OutputSizes=1,1
  Selector19 : Selector  NumberOfDimensions=2  InputPortWidth=3  IndexOptions=Index vector (dialog),Index vector (dialog)  Indices=2,[1 2 3]  OutputSizes=1,1
  Selector20 : Selector  NumberOfDimensions=2  InputPortWidth=3  IndexOptions=Index vector (dialog),Index vector (dialog)  Indices=3,[1 2 3]  OutputSizes=1,1
  Selector21 : Selector  InputPortWidth=10  IndexOptions=Index vector (dialog)  Indices=[7 8 9 10]  OutputSizes=1
  Sum : Sum  Inputs=+-
  Sum of Elements : Sum  Inputs=+  CollapseMode=Specified dimension  CollapseDim=2
  Sum1 : Sum
  Sum{10..13} (4 alike) : Sum  Inputs=|+|+|
  Sum3 : Sum  Inputs=+-
  Sum4 : Sum
  Terminator : Terminator
  Terminator3 : Terminator
  Transpose : Math  Operator=transpose  SaturateOnIntegerOverflow=on
  Vector Concatenate2 : Concatenate  NumInputs=4
  Vector Concatenate3 : Concatenate  NumInputs=4
  Vector Concatenate6 : Concatenate  NumInputs=6
  creation of the areas of the S/C : Subsystem
  F_MB : Outport
  F_SP : Outport  Port=2
  A_MB : Outport  Port=3
  prodsca_MB : Outport  Port=4
  prodscal_SP : Outport  Port=5
  wires:
  Gain/1 -> Product/1
  Reshape9/1 -> prodscal_SP/1, Product6/1, Matrix Multiply2/1
  Gain5/1 -> Product6/2
  Constant1/1 -> Sum3/1
  Gain1/1 -> Product2/2
  Reshape5/1 -> [RD_SP]
  SB/1 -> Transpose/1
  Add/1 -> Product/4
  Gain6/1 -> Sum4/2
  Gain4/1 -> Product4/1
  [P] -> Gain/1
  Reshape4/1 -> [RD_MB]
  Sum3/1 -> Product5/2
  Product6/1 -> Sum4/1
  Constant5/1 -> Sum3/2, Gain5/1
  Product2/1 -> Sum1/1
  [RD_MB] -> Gain2/1
  Gain2/1 -> Sum1/2
  Constant/1 -> Sum/1
  Constant4/1 -> Sum/2, Gain1/1
  Sum/1 -> Product1/2
  Product/1 -> F_MB/1
  [P] -> Gain4/1
  [RD_SP] -> Gain6/1
  Constant6/1 -> Product8/1
  Product8/1 -> [P]
  [S_B] -> Product1/1
  Constant8/1 -> Reshape2/1
  Reshape2/1 -> Matrix Multiply/2
  Sum1/1 -> Matrix Multiply/1
  Matrix Multiply/1 -> Product3/2
  Constant9/1 -> Reshape1/1
  Reshape1/1 -> Matrix Multiply1/2
  Matrix Multiply1/1 -> Product/3
  Transpose/1 -> [S_B]
  Selector14/1 -> Dot Product7/2
  [S_B] -> Dot Product8/1
  Selector15/1 -> Dot Product8/2
  Selector16/1 -> Dot Product9/2
  [S_B] -> Dot Product7/1
  [S_B] -> Dot Product1/1
  Dot Product8/1 -> Vector Concatenate2/3
  Dot Product7/1 -> Vector Concatenate2/2
  Dot Product1/1 -> Vector Concatenate2/1
  Dot Product9/1 -> Vector Concatenate2/4
  Selector13/1 -> Dot Product1/2
  N_SP/1 -> Selector13/1, Selector14/1, Product7/1, Selector16/1, Selector15/1
  [S_B] -> Dot Product9/1
  Reshape3/1 -> Matrix Multiply2/2
  Constant12/1 -> Reshape3/1
  Matrix Multiply2/1 -> Product4/3
  [S_B] -> Product5/1
  Constant13/1 -> Reshape6/1
  Reshape6/1 -> Matrix Multiply3/2
  Sum4/1 -> Matrix Multiply3/1
  Matrix Multiply3/1 -> Product7/2
  Selector20/1 -> Sum12/2
  Sum13/1 -> Vector Concatenate3/4
  Selector19/1 -> Sum11/2
  Selector18/1 -> Sum10/2
  Sum10/1 -> Vector Concatenate3/1
  Sum12/1 -> Vector Concatenate3/3
  Sum11/1 -> Vector Concatenate3/2
  Product7/1 -> Selector17/1, Selector20/1, Selector18/1, Selector19/1
  Selector17/1 -> Sum13/2
  Product5/1 -> Sum10/1, Sum11/1, Sum13/1, Sum12/1
  Reshape10/1 -> Product4/4
  Reshape7/1 -> Matrix Multiply4/2
  Constant14/1 -> Reshape7/1
  Matrix Multiply4/1 -> Product/2
  Reciprocal/1 -> Product8/2
  Constant7/1 -> Reciprocal/1
  Vector Concatenate2/1 -> Reshape9/1
  Vector Concatenate3/1 -> Reshape10/1
  Product4/1 -> F_SP/1
  Vector Concatenate6/1 -> Reshape14/1
  creation of the areas of the S/C/1(a*b_1) -> Vector Concatenate6/1
  creation of the areas of the S/C/2(a*b_2) -> Vector Concatenate6/2
  creation of the areas of the S/C/3(a*h_1) -> Vector Concatenate6/3
  creation of the areas of the S/C/4(a*h_2) -> Vector Concatenate6/4
  creation of the areas of the S/C/5(b*h_1) -> Vector Concatenate6/5
  creation of the areas of the S/C/6(b*h_2) -> Vector Concatenate6/6
  Reshape14/1 -> A_MB/1, Matrix Multiply4/1
  MB/1 -> [MB]
  SP/1 -> Demux/1
  Demux/2 -> [a_SP]
  Demux/4 -> Terminator3/1
  Demux/3 -> [b_SP]
  Demux/1 -> Terminator/1
  [a_SP] -> Product9/1
  [b_SP] -> Product9/2
  Product9/1 -> Product4/2
  Selector/1 -> Reshape4/1
  Selector21/1 -> Reshape5/1
  Constant2/1 -> Selector21/1, Selector/1
  [MB] -> creation of the areas of the S/C/1(MB)
  Constant3/1 -> Reshape11/1
  Reshape11/1 -> Matrix Multiply5/1
  Matrix Multiply5/1 -> Product10/1
  Product10/1 -> Sum of Elements/1
  [S_B] -> Reshape12/1
  Reshape12/1 -> Matrix Multiply5/2
  N_MB/1 -> [N_MB]
  [N_MB] -> Product3/1
  [N_MB] -> Product10/2
  Sum of Elements/1 -> [dot_N_MB_SB]
  [dot_N_MB_SB] -> Matrix Multiply1/1
  [dot_N_MB_SB] -> Product2/1
  Constant10/1 -> Reshape/1
  Reshape/1 -> Matrix Multiply6/1
  Product1/1 -> Matrix Multiply6/2
  Matrix Multiply6/1 -> Add/1
  Product3/1 -> Add/2
  [dot_N_MB_SB] -> prodsca_MB/1

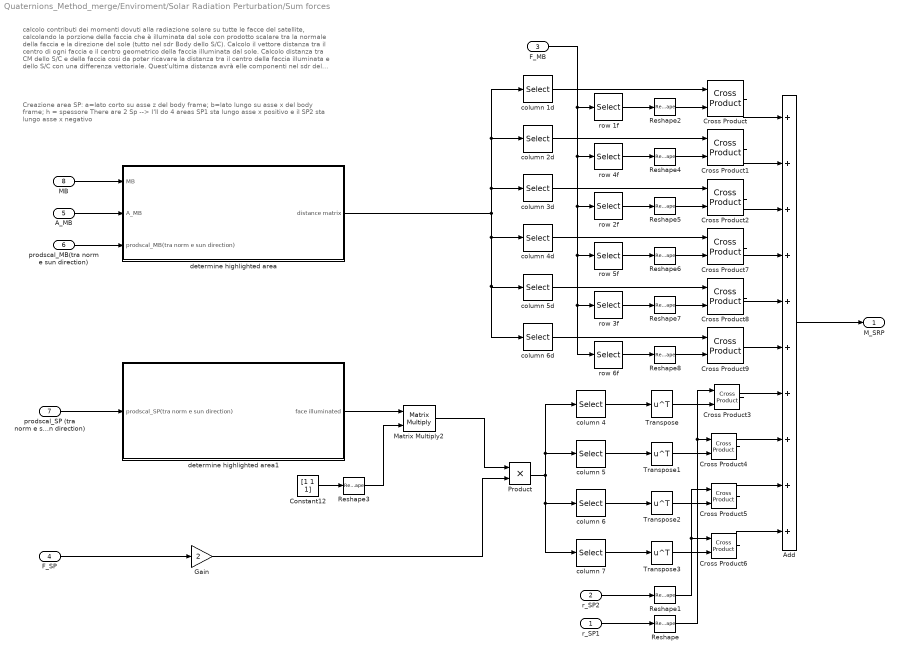
== system Quaternions_Method_merge/Enviroment/Solar Radiation Perturbation/Sum forces ==
  note: Creazione area SP: a=lato corto su asse z del body frame; b=lato lungo su asse x del body frame; h = spessore
      | There are 2 Sp --> I'll do 4 areas
      | SP1 sta lungo asse x positivo e il SP2 sta lungo asse x negativo
  note: calcolo contributi dei momenti dovuti alla radiazione solare su tutte le facce del satellite, calcolando la porzione della faccia che è illuminata dal sole con prodotto scalare tra la normale della faccia e la direzione del sole (tutto nel sdr Body dello S/C). Calcolo il vettore distanza tra il centro di ogni faccia e il centro geometrico della faccia illuminata dal sole. Calcolo distanza tra CM dello S/C e della faccia cosi da poter ricavare la distanza tra il centro della faccia illuminata e dello S/C con una differenza vettoriale. Quest'ultima distanza avrà elle componenti nel sdr del S/C (body)
  r_SP1 : Inport
  r_SP2 : Inport  Port=2
  F_MB : Inport  Port=3
  F_SP : Inport  Port=4
  A_MB : Inport  Port=5
  prodscal_MB(tra norm e sun direction) : Inport  Port=6
  prodscal_SP (tra norm e sun direction) : Inport  Port=7
  MB : Inport  Port=8
  Add : Sum  Inputs=+|+|+|+|+|+|+|+|+|+
  Constant12 : Constant  Value=[1 1 1]
  Cross Product{,1..9} (10 alike) : matrix_library/Cross Product
      settings: SourceProductBaseCode=SL
  Gain : Gain  Gain=2
  Matrix Multiply2 : Product  Multiplication=Matrix(*)
  Product : Product
  Reshape{,1..2,4..8} (8 alike) : Reshape  OutputDimensionality=Column vector (2-D)
  Reshape3 : Reshape  OutputDimensionality=Row vector (2-D)
  Transpose{,1..3} (4 alike) : Math  Operator=transpose  SaturateOnIntegerOverflow=on
  column 1d : Selector  NumberOfDimensions=2  InputPortWidth=3  IndexOptions=Index vector (dialog),Index vector (dialog)  Indices=[1 2 3],1  OutputSizes=1,1
  column 2d : Selector  NumberOfDimensions=2  InputPortWidth=3  IndexOptions=Index vector (dialog),Index vector (dialog)  Indices=[1 2 3],2  OutputSizes=1,1
  column 3d : Selector  NumberOfDimensions=2  InputPortWidth=3  IndexOptions=Index vector (dialog),Index vector (dialog)  Indices=[1 2 3],3  OutputSizes=1,1
  column 4 : Selector  NumberOfDimensions=2  InputPortWidth=3  IndexOptions=Index vector (dialog),Index vector (dialog)  Indices=1,[1 2 3]  OutputSizes=1,1
  column 4d : Selector  NumberOfDimensions=2  InputPortWidth=3  IndexOptions=Index vector (dialog),Index vector (dialog)  Indices=[1 2 3],1  OutputSizes=1,1
  column 5 : Selector  NumberOfDimensions=2  InputPortWidth=3  IndexOptions=Index vector (dialog),Index vector (dialog)  Indices=2,[1 2 3]  OutputSizes=1,1
  column 5d : Selector  NumberOfDimensions=2  InputPortWidth=3  IndexOptions=Index vector (dialog),Index vector (dialog)  Indices=[1 2 3],2  OutputSizes=1,1
  column 6 : Selector  NumberOfDimensions=2  InputPortWidth=3  IndexOptions=Index vector (dialog),Index vector (dialog)  Indices=3,[1 2 3]  OutputSizes=1,1
  column 6d : Selector  NumberOfDimensions=2  InputPortWidth=3  IndexOptions=Index vector (dialog),Index vector (dialog)  Indices=[1 2 3],3  OutputSizes=1,1
  column 7 : Selector  NumberOfDimensions=2  InputPortWidth=3  IndexOptions=Index vector (dialog),Index vector (dialog)  Indices=4,[1 2 3]  OutputSizes=1,1
  determine highlighted area : Subsystem
  determine highlighted area1 : Subsystem
  row 1f : Selector  NumberOfDimensions=2  InputPortWidth=3  IndexOptions=Index vector (dialog),Index vector (dialog)  Indices=1,[1 2 3]  OutputSizes=1,1
  row 2f : Selector  NumberOfDimensions=2  InputPortWidth=3  IndexOptions=Index vector (dialog),Index vector (dialog)  Indices=2,[1 2 3]  OutputSizes=1,1
  row 3f : Selector  NumberOfDimensions=2  InputPortWidth=3  IndexOptions=Index vector (dialog),Index vector (dialog)  Indices=3,[1 2 3]  OutputSizes=1,1
  row 4f : Selector  NumberOfDimensions=2  InputPortWidth=3  IndexOptions=Index vector (dialog),Index vector (dialog)  Indices=4,[1 2 3]  OutputSizes=1,1
  row 5f : Selector  NumberOfDimensions=2  InputPortWidth=3  IndexOptions=Index vector (dialog),Index vector (dialog)  Indices=5,[1 2 3]  OutputSizes=1,1
  row 6f : Selector  NumberOfDimensions=2  InputPortWidth=3  IndexOptions=Index vector (dialog),Index vector (dialog)  Indices=6,[1 2 3]  OutputSizes=1,1
  M_SRP : Outport
  wires:
  prodscal_MB(tra norm e sun direction)/1 -> determine highlighted area/3(prodscal_MB(tra norm e sun direction))
  Add/1 -> M_SRP/1
  A_MB/1 -> determine highlighted area/2(A_MB)
  column 2d/1 -> Cross Product1/1
  column 1d/1 -> Cross Product/1
  column 3d/1 -> Cross Product2/1
  Cross Product1/1 -> Add/2
  Cross Product/1 -> Add/1
  Cross Product2/1 -> Add/3
  prodscal_SP (tra norm e sun direction)/1 -> determine highlighted area1/1(prodscal_SP(tra norm e sun direction))
  F_SP/1 -> Gain/1
  Gain/1 -> Product/2
  Reshape3/1 -> Matrix Multiply2/2
  Constant12/1 -> Reshape3/1
  determine highlighted area1/1(face illuminated) -> Matrix Multiply2/1
  Matrix Multiply2/1 -> Product/1
  r_SP1/1 -> Reshape/1
  r_SP2/1 -> Reshape1/1
  Product/1 -> column 7/1, column 6/1, column 4/1, column 5/1
  Cross Product3/1 -> Add/7
  Cross Product4/1 -> Add/8
  Cross Product5/1 -> Add/9
  Cross Product6/1 -> Add/10
  column 4/1 -> Transpose/1
  column 5/1 -> Transpose1/1
  column 6/1 -> Transpose2/1
  column 7/1 -> Transpose3/1
  Reshape/1 -> Cross Product3/1, Cross Product4/1
  Reshape1/1 -> Cross Product5/1, Cross Product6/1
  Transpose/1 -> Cross Product3/2
  Transpose1/1 -> Cross Product4/2
  Transpose2/1 -> Cross Product5/2
  Transpose3/1 -> Cross Product6/2
  Cross Product9/1 -> Add/6
  Cross Product7/1 -> Add/4
  Cross Product8/1 -> Add/5
  column 6d/1 -> Cross Product9/1
  column 4d/1 -> Cross Product7/1
  column 5d/1 -> Cross Product8/1
  determine highlighted area/1(distance matrix) -> column 2d/1, column 1d/1, column 3d/1, column 6d/1, column 5d/1, column 4d/1
  row 1f/1 -> Reshape2/1
  row 4f/1 -> Reshape4/1
  row 2f/1 -> Reshape5/1
  row 5f/1 -> Reshape6/1
  row 3f/1 -> Reshape7/1
  row 6f/1 -> Reshape8/1
  F_MB/1 -> row 6f/1, row 3f/1, row 5f/1, row 2f/1, row 4f/1, row 1f/1
  Reshape2/1 -> Cross Product/2
  Reshape4/1 -> Cross Product1/2
  Reshape5/1 -> Cross Product2/2
  Reshape6/1 -> Cross Product7/2
  Reshape7/1 -> Cross Product8/2
  Reshape8/1 -> Cross Product9/2
  MB/1 -> determine highlighted area/1(MB)

== system Quaternions_Method_merge/Enviroment/Solar Radiation Perturbation/Sun position body ==
  A_B_N : Inport
  Clock : Clock
  Constant : Constant  Value=2*pi
  Constant1 : Constant  Value=365*24*60*60
  Constant2 : Constant  Value=23.45
  Degrees to Radians : simulink_extras/Transformations/Degrees to Radians
  MatrixMultiply : Product  Multiplication=Matrix(*)
  Mux : Mux  Inputs=3
  Product{,1..3} (4 alike) : Product
  Reciprocal : Product  Inputs=1
  Reshape : Reshape  OutputDimensionality=Column vector (2-D)
  Sin : Trigonometry  Operator=cos
  Sin1 : Trigonometry
  Sin2 : Trigonometry  Operator=cos
  Sin3 : Trigonometry
  S_B : Outport
  wires:
  Product3/1 -> Mux/3
  Degrees to Radians/1 -> Sin3/1, Sin2/1
  Constant1/1 -> Reciprocal/1
  Sin2/1 -> Product2/2
  Product/1 -> Product1/1  "n"
  Constant2/1 -> Degrees to Radians/1
  Product1/1 -> Sin/1, Sin1/1  "n*t"
  Product2/1 -> Mux/2
  Sin3/1 -> Product3/2
  Clock/1 -> Product1/2
  Sin1/1 -> Product3/1, Product2/1
  Constant/1 -> Product/1
  Sin/1 -> Mux/1
  Reciprocal/1 -> Product/2
  Mux/1 -> Reshape/1
  A_B_N/1 -> MatrixMultiply/1
  MatrixMultiply/1 -> S_B/1
  Reshape/1 -> MatrixMultiply/2

== system Quaternions_Method_merge/Kinematics/Creazione Matrice A_BN/column 1 ==
  q_normalizzato : Inport
  Demux : Demux
  Gain : Gain  Gain=2
  Gain1 : Gain  Gain=2
  Mux : Mux  Inputs=3
  Product{,1..3} (4 alike) : Product
  Square{,1..3} (4 alike) : Math  Operator=square  SaturateOnIntegerOverflow=on
  Sum : Sum  Inputs=|+|-|-|+|
  Sum1 : Sum  Inputs=|+|-|
  Sum2 : Sum  Inputs=|+|+|
  Column 1 : Outport
  wires:
  Demux/4 -> [q4]
  Demux/1 -> [q1]
  q_normalizzato/1 -> Demux/1
  Demux/3 -> [q3]
  Demux/2 -> [q2]
  [q1] -> Square/1
  [q2] -> Square3/1
  [q3] -> Square2/1
  [q4] -> Square1/1
  Square3/1 -> Sum/2
  Square/1 -> Sum/1
  Square1/1 -> Sum/4
  Square2/1 -> Sum/3
  [q4] -> Product1/2
  [q1] -> Product/1
  [q2] -> Product/2
  [q3] -> Product1/1
  Product/1 -> Sum1/1
  Product1/1 -> Sum1/2
  Sum1/1 -> Gain/1
  [q4] -> Product3/2
  [q1] -> Product2/1
  Product3/1 -> Sum2/2
  Product2/1 -> Sum2/1
  Sum2/1 -> Gain1/1
  [q3] -> Product2/2
  [q2] -> Product3/1
  Sum/1 -> Mux/1
  Gain/1 -> Mux/2
  Gain1/1 -> Mux/3
  Mux/1 -> Column 1/1

== system Quaternions_Method_merge/Kinematics/Creazione Matrice A_BN/column 2 ==
  q_normalizzato : Inport
  Demux : Demux
  Gain : Gain  Gain=2
  Gain1 : Gain  Gain=2
  Mux : Mux  Inputs=3
  Product{,1..3} (4 alike) : Product
  Square{,1..3} (4 alike) : Math  Operator=square  SaturateOnIntegerOverflow=on
  Sum : Sum  Inputs=|-|+|-|+|
  Sum1 : Sum  Inputs=|+|+|
  Sum2 : Sum  Inputs=|+|-|
  Column 2 : Outport
  wires:
  Demux/4 -> [q4]
  Demux/1 -> [q1]
  q_normalizzato/1 -> Demux/1
  Demux/3 -> [q3]
  Demux/2 -> [q2]
  Mux/1 -> Column 2/1
  Gain1/1 -> Mux/3
  Product2/1 -> Sum2/1
  Product3/1 -> Sum2/2
  Sum2/1 -> Gain1/1
  Sum1/1 -> Gain/1
  [q2] -> Product/2
  [q3] -> Product1/1
  [q4] -> Product1/2
  Product/1 -> Sum1/1
  Gain/1 -> Mux/1
  [q1] -> Product/1
  Product1/1 -> Sum1/2
  Sum/1 -> Mux/2
  [q1] -> Square/1
  Square1/1 -> Sum/4
  Square3/1 -> Sum/2
  [q4] -> Square1/1
  Square2/1 -> Sum/3
  [q2] -> Square3/1
  [q3] -> Square2/1
  Square/1 -> Sum/1
  [q2] -> Product2/1
  [q3] -> Product2/2
  [q1] -> Product3/1
  [q4] -> Product3/2

== system Quaternions_Method_merge/Kinematics/Creazione Matrice A_BN/column 3 ==
  q_normalizzato : Inport
  Demux : Demux
  Gain : Gain  Gain=2
  Gain1 : Gain  Gain=2
  Mux : Mux  Inputs=3
  Product{,1..3} (4 alike) : Product
  Square{,1..3} (4 alike) : Math  Operator=square  SaturateOnIntegerOverflow=on
  Sum : Sum  Inputs=|-|-|+|+|
  Sum1 : Sum  Inputs=|+|-|
  Sum2 : Sum  Inputs=|+|+|
  Column 3 : Outport
  wires:
  Demux/4 -> [q4]
  Demux/1 -> [q1]
  q_normalizzato/1 -> Demux/1
  Demux/3 -> [q3]
  Demux/2 -> [q2]
  Gain/1 -> Mux/1
  Product1/1 -> Sum1/2
  [q4] -> Product1/2
  Product/1 -> Sum1/1
  Mux/1 -> Column 3/1
  [q1] -> Product/1
  Sum1/1 -> Gain/1
  [q1] -> Square/1
  Square2/1 -> Sum/3
  Square3/1 -> Sum/2
  [q4] -> Square1/1
  Square1/1 -> Sum/4
  Square/1 -> Sum/1
  Sum/1 -> Mux/3
  [q3] -> Square2/1
  [q2] -> Square3/1
  [q2] -> Product2/1
  Product3/1 -> Sum2/2
  Gain1/1 -> Mux/2
  Sum2/1 -> Gain1/1
  Product2/1 -> Sum2/1
  [q3] -> Product2/2
  [q4] -> Product3/2
  [q1] -> Product3/1
  [q3] -> Product/2
  [q2] -> Product1/1
